simulink model "pwm"  (R2013a)
settings: Solver=ode45  StartTime=0.0  StopTime=3  RelTol=1e-3
libraries: powerlib x1
settings Model: Creator=SHAHID  LastModifiedBy=Sunny
settings DataIOCC: SignalLoggingSaveFormat=ModelDataLogs
settings OptimizationCC: ExpressionDepthLimit=2147483647
settings DebuggingCC: FcnCallInpInsideContextMsg=UseLocalSettings
settings GRTTargetCC: CombineOutputUpdateFcns=off  GRTInterface=on

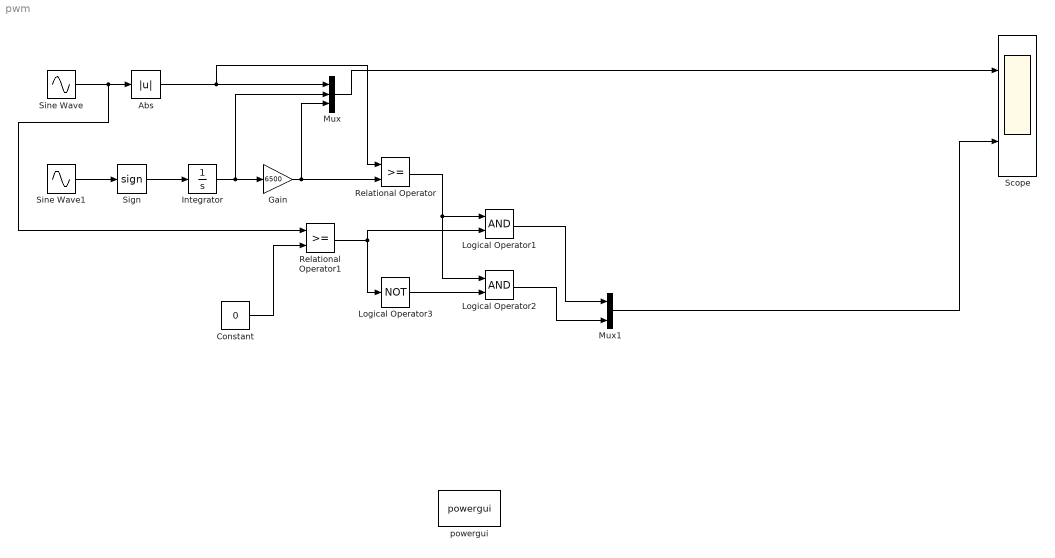
== system pwm ==
  Abs : Abs
  Constant : Constant  Value=0
  Gain : Gain  Gain=6500
  Integrator : Integrator
  Logical Operator1 : Logic  AllPortsSameDT=off  OutDataTypeStr=boolean
  Logical Operator2 : Logic  AllPortsSameDT=off  OutDataTypeStr=boolean
  Logical Operator3 : Logic  Operator=NOT  AllPortsSameDT=off  OutDataTypeStr=boolean
  Mux : Mux  Inputs=3
  Mux1 : Mux  Inputs=2
  Relational Operator : RelationalOperator  InputSameDT=on
  Relational Operator1 : RelationalOperator  InputSameDT=on
  Scope : Scope  NumInputPorts=2
      settings: TimeRange=0.5  YMin=-0.1~-5  YMax=2.1~5  MaxDataPoints=500
  Sign : Signum
  Sine Wave : Sin  Frequency=2*pi*50  SampleTime=0
  Sine Wave1 : Sin  Frequency=2*pi*3000  SampleTime=0
  powergui : powerlib/powergui  Priority=1  SimulationMode=Continuous  SolverType=Tustin  SampleTime=50e-6  frequency=60  SPID=off  DisableSnubberDevices=off  DisableRonSwitches=off  DisableVfSwitches=off  SwTol=0  Interpol=off  DisplayEquations=off  frequencyindice=0  Pbase=100e6  ErrMax=1e-4  Iterations=50  UnitsV=kV  UnitsW=MW  FunctionMessages=off  echomessages=off  HookPort=off  EnableUseOfTLC=off  x0status=steady  RestoreLinks=no  ResistiveCurrentMeasurement=off  Frange=[0:2:500]  Ylog=off  Xlog=on  ShowGrid=off  save=off  variable=ZData  structure=ScopeData8  ZoomFFT=off  StartTime=0.0  cycles=1  DisplayStyle=1  fundamental=60  FreqAxis=off  MaxFrequency=1000  frequencyindicesteady=1  RmsSteady=1  display=off  Ts=0  methode=off
  wires:
  Sine Wave/1 -> Abs/1, Relational Operator1/1
  Abs/1 -> Mux/1, Relational Operator/1
  Sine Wave1/1 -> Sign/1
  Sign/1 -> Integrator/1
  Integrator/1 -> Mux/2, Gain/1
  Gain/1 -> Mux/3, Relational Operator/2
  Logical Operator3/1 -> Logical Operator2/2
  Mux1/1 -> Scope/2
  Relational Operator/1 -> Logical Operator1/1, Logical Operator2/1
  Logical Operator1/1 -> Mux1/1
  Logical Operator2/1 -> Mux1/2
  Constant/1 -> Relational Operator1/2
  Relational Operator1/1 -> Logical Operator3/1, Logical Operator1/2
  Mux/1 -> Scope/1
